simulink model "Final_Battery_model (1)"  (R2023b)
settings: Solver=VariableStepAuto  StartTime=0.0  StopTime=inf  FixedStep=1  RelTol=1e-5
undefined symbols (not defined in the file): C
settings Model: PacingRate=100  Creator=vahid  LastModifiedBy=vahid
settings SolverCC: ZeroCrossAlgorithm=Adaptive
settings OptimizationCC: BlockReduction=off  DefaultParameterBehavior=Inlined  BufferReuse=off
settings DebuggingCC: IgnoredZcDiagnostic=none

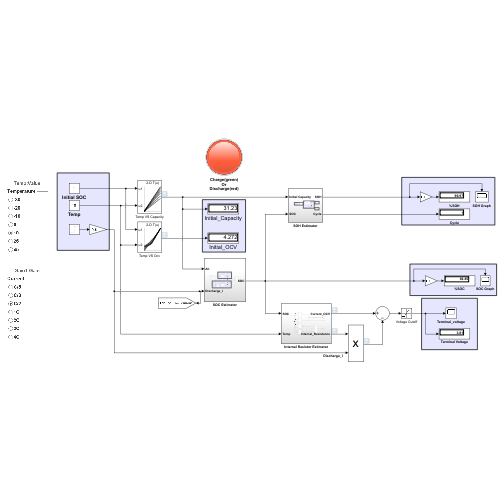
[thumbnail: Simulink's stored preview of the top-level diagram]
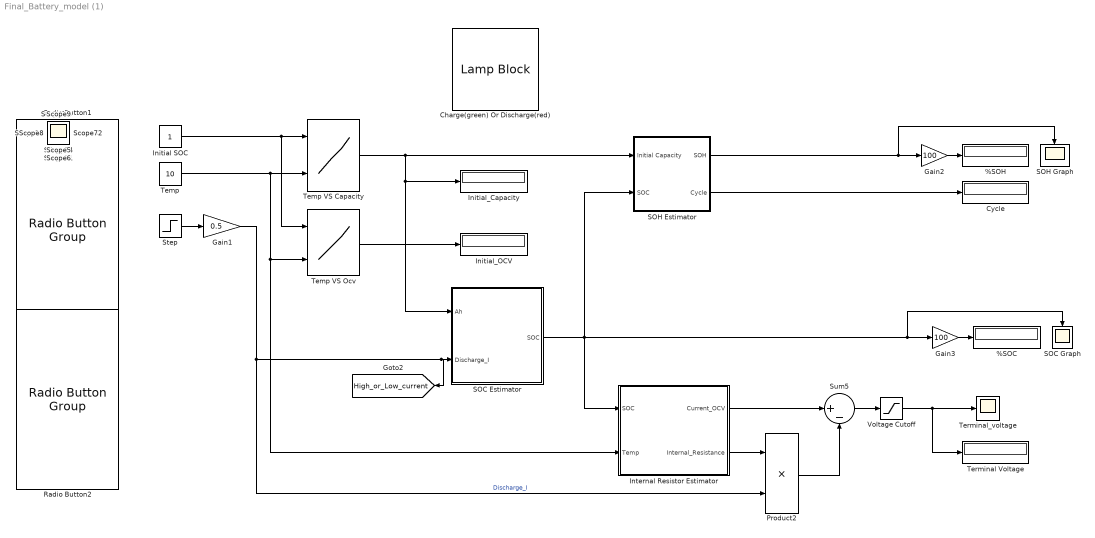
== system Final_Battery_model (1) ==
  %SOC : Display
  %SOH : Display
  Charge(green) Or Discharge(red) : LampBlock  LabelPosition=Hide
  Cycle : Display
  Gain1 : Gain  Gain=0.5
  Gain2 : Gain  Gain=100
  Gain3 : Gain  Gain=100
  Initial SOC : Constant  SampleTime=1
  Initial_Capacity : Display
  Initial_OCV : Display
  Internal Resistor Estimator : Subsystem
  Product2 : Product
  Radio Button1 : RadioButtonGroup  SelectedLabel=10  ButtonGroupName=Temperature
      settings: Values={{'-30', '-20', '-10', '0', '10', '25', '45'}, [-30 -20 -10 0 10 25 45]}
  Radio Button2 : RadioButtonGroup  SelectedLabel=C/2  ButtonGroupName=Current
      settings: Values={{'C/5', 'C/3', 'C/2', '1C', '2C', '3C', '4C'}, [0.2 0.33 0.5 1 2 3 4]}
  SOC Estimator : Subsystem
  SOC Graph : Scope
  SOH Estimator : Subsystem
  SOH Graph : Scope
  Step : Step  Before=32  After=32  SampleTime=0
  Sum5 : Sum  Inputs=|+-
  Temp : Constant  Value=10
  Temp VS Capacity : Lookup_n-D  BreakpointsForDimension1=[0.05;0.1;0.2;0.3;0.4;0.5;0.6;0.7;0.8;0.9;1]  BreakpointsForDimension2=[-30;-20;-10;0;10;25;45;55]  Table=[0.9696 1.142325 1.332525 1.44755 1.561325 1.666425 1.751575 1.7742;1.9392 2.28465 2.66505 2.8951 3.12265 3.33285 3.50315 3.5484;3.8784 4.5693 5.3301 5.7902 6.2453 6.6657 7.0063 7.0968;5.8176 6.85395 7.99515 8.6853 9.36795 9.99855 10.50945 10.6452;7.7568 9.1386 10.6602 11.5804 12.4906 13.3314 14.0126 14.1936;9.696 11.42325 13.32525 14.4755 15.61325 16.66425 17.51575 17.742;11.6352 13.7079 15.9903 17.3706 18.7359 19.9971 21.0189 21.2904;13.5744 15.99255 18.65535 20.2657 21.85855 23.32995 24.52205 24.8388;15.5136 18.2772 21.3204 23.1608 24.9812 26.6628 28.0252 28.3872;17.4528 20.56185 23.98545 26.0559 28.10385 29.99565 31.52835 31.9356;19.392 22.8465 26.6505 28.951 31.2265 33.3285 35.0315 35.484]  InternalRulePriority=Speed  RndMeth=Simplest
      settings: InputPortMap=u0,u1
  Temp VS Ocv : Lookup_n-D  BreakpointsForDimension1=[0.05;0.1;0.2;0.3;0.4;0.5;0.6;0.7;0.8;0.9;1]  BreakpointsForDimension2=[-30;-20;-10;0;10;25;45;55]  Table=[3.631 3.597 3.574 3.559 3.523 3.473 3.473 3.425;3.635 3.61 3.588 3.581 3.558 3.516 3.516 3.462;3.669 3.647 3.625 3.617 3.608 3.589 3.589 3.547;3.713 3.69 3.663 3.651 3.641 3.632 3.632 3.619;3.768 3.749 3.715 3.694 3.678 3.665 3.665 3.655;3.831 3.821 3.788 3.764 3.743 3.72 3.72 3.702;3.898 3.901 3.878 3.862 3.85 3.831 3.831 3.806;3.971 3.984 3.973 3.968 3.957 3.938 3.938 3.917;4.048 4.071 4.069 4.07 4.063 4.05 4.05 4.033;4.133 4.154 4.158 4.165 4.164 4.161 4.161 4.149;4.266 4.268 4.266 4.272 4.272 4.278 4.278 4.261]  InternalRulePriority=Speed  RndMeth=Simplest
      settings: InputPortMap=u0,u1
  Terminal Voltage : Display
  Terminal_voltage : Scope
  Voltage Cutoff : Saturate  UpperLimit=4.3  LowerLimit=2.7
  Scope{,2..15} (15 alike) : Scope
  tag scope: High_or_Low_current=global
  wires:
  Temp VS Capacity/1 -> SOH Estimator/1(Initial Capacity), Initial_Capacity/1, SOC Estimator/1(Ah)
  Temp VS Ocv/1 -> Initial_OCV/1
  Initial SOC/1 -> Temp VS Ocv/1, Temp VS Capacity/1
  Temp/1 -> Internal Resistor Estimator/2(Temp), Temp VS Ocv/2, Temp VS Capacity/2
  Product2/1 -> Sum5/2
  Internal Resistor Estimator/1(Current_OCV) -> Sum5/1
  Internal Resistor Estimator/2(Internal_Resistance) -> Product2/1
  Step/1 -> Gain1/1
  Gain1/1 -> [High_or_Low_current], SOC Estimator/2(Discharge_I), Product2/2  "Discharge_I"
  Sum5/1 -> Voltage Cutoff/1
  SOH Estimator/1(SOH) -> SOH Graph/1, Gain2/1
  Gain2/1 -> %SOH/1
  SOH Estimator/2(Cycle) -> Cycle/1
  SOC Estimator/1(SOC) -> Internal Resistor Estimator/1(SOC), Gain3/1, SOC Graph/1, SOH Estimator/2(SOC)
  Voltage Cutoff/1 -> Terminal Voltage/1, Terminal_voltage/1
  Gain3/1 -> %SOC/1

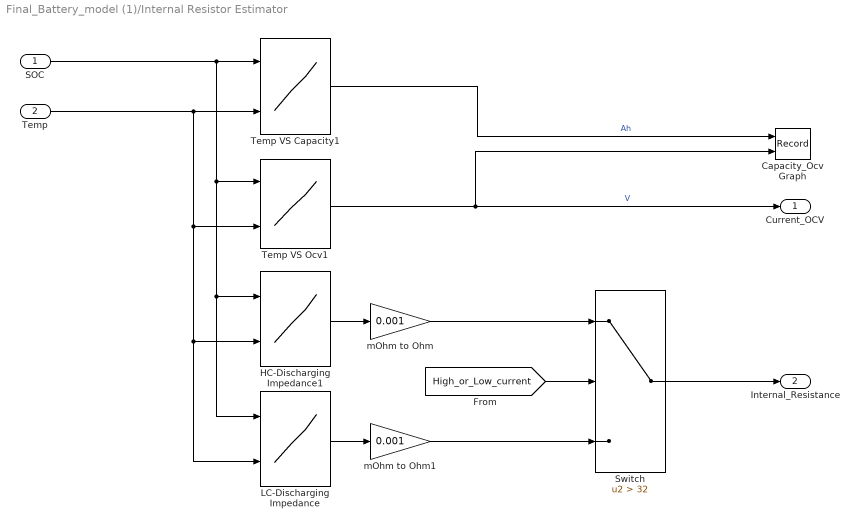
== system Final_Battery_model (1)/Internal Resistor Estimator ==
  SOC : Inport
  Temp : Inport  Port=2
  Capacity_Ocv Graph : Record  FileSettingsInternal="{\"entries\":[{\"content\":{\"excelSettings\":{\"content\":{},\"type\":\"Streamout.ExcelSettings\"}},\"type\":\"Streamout.FileSettingStorage\",\"uuid\":\"\"}],\"packageUris\":[\"http:\\/\\/schema.mathworks.com\\/mf0\\/streamout_blocks\\/R2020a\"],\"version\":\"1.0\"}"  Layout=[1 1]  SignalsInternal="{\"entries\":[{\"content\":{\"signals\":[{\"content\":{\"blockPath\":[],\"dimensions\":[1],\"domain\":\"\",\"lineColor\":\"#a2142f\",\"plots\":[1],\"port\":1,\"signalID\":7779,\"signalName\":\"XY Graph:1\"},\"type\":\"RecordBlkView.Signal\",\"uuid\":\"\"},{\"content\":{\"blockPath\":[],\"dimensions\":[1],\"domain\":\"\",\"lineColor\":\"#139fff\",\"plots\":[1],\"port\":2,\"signalID\":7782,\"signalName\":\"XY Graph:2\"},\"type\":\"RecordBlkView.Signal\",\"uuid\":\"\"}]},\"type\":\"RecordBlkView.InputSignals\",\"uuid\":\"\"}],\"packageUris\":[\"http:\\/\\/schema.mathworks.com\\/mf0\\/streamout_blocks\\/R2020a\"],\"version\":\"1.0\"}"  VisualizationBindings="{\"xyplotplugin\":{\"info\":[{\"series\":[{\"bindingParametersList\":[{\"parameter\":\"X-Axis\",\"signalID\":7779,\"signalName\":\"XY Graph:1\"},{\"parameter\":\"Y-Axis\",\"signalID\":7782,\"signalName\":\"XY Graph:2\"}],\"seriesID\":9451}],\"subplotID\":1}]}}"  CompatibilityTag=XY
  HC-Discharging Impedance1 : Lookup_n-D  BreakpointsForDimension1=[0;0.05;0.1;0.2;0.3;0.4;0.5;0.6;0.7;0.8;0.9;1]  BreakpointsForDimension2=[-30;-20;-10;0;10;25;45;55]  Table=[75.5 51.2 28.1 17.5 14.1 8.88 5.49 4.87;75.5 51.2 28.1 17.5 14.1 8.88 5.49 4.87;69.9 45.3 24.1 14.2 10.3 7.3 3.2 4.2;61.2 35.8 17.8 10 6.1 4.3 3.5 2.3;47.7 26.6 13.8 8.1 5.1 4 3 2;37.1 23.5 11.7 7.4 4.8 3.7 3 1.9;30.5 21.4 10.6 7.1 4.7 3.9 2.2 1.7;27.5 18.3 10 7 4.7 3.9 2.1 1.7;24.8 16.7 9.7 6.9 4.7 4 2.2 1.9;22.9 16.1 9.5 6.9 4.8 4 2.3 1.9;22.1 15.8 9.5 7 4.9 4.1 2.3 1.9;22.4 16.7 9.7 7.3 5.1 3.9 2.2 1.8]  InternalRulePriority=Speed  RndMeth=Simplest
      settings: InputPortMap=u0,u1
  LC-Discharging Impedance : Lookup_n-D  BreakpointsForDimension1=[0;0.05;0.1;0.15;0.2;0.25;0.3;0.35;0.4;0.45;0.5;0.55;0.6;0.65;0.7;0.75;0.8;0.85;0.9;0.95;1]  BreakpointsForDimension2=[-30;-20;-10;0;10;25;45]  Table=[124.53 60.78 33.59 13.67 8.39 4.69 3.13;124.53 60.78 33.59 13.67 8.39 4.69 3.13;122.03 59.69 32.5 12.61 7.28 3.91 2.34;119.84 58.59 31.88 11.97 6.78 3.44 2.03;119.38 57.5 30.94 11.54 6.51 3.28 1.87;118.59 56.41 30.31 11.27 6.32 3.28 1.88;117.97 55.78 29.84 11.17 6.2 2.97 1.87;117.34 55.63 29.53 11.05 6.13 3.13 1.88;117.03 55.63 29.38 11.08 6.22 3.12 1.72;116.88 55.62 29.53 11.22 6.3 3.28 1.88;116.72 55.78 29.69 11.51 6.49 3.28 1.88;117.03 55.78 30 11.78 6.75 3.59 2.03;117.19 55.94 30 12.04 7.14 3.91 2.19;117.34 56.41 30.16 12.21 7.11 3.75 2.19;118.28 57.03 30.47 12.3 7.09 3.75 2.19;119.53 57.81 30.94 12.42 7.09 3.91 2.19;121.56 59.06 31.25 12.42 7.18 3.59 2.19;124.38 60.47 31.88 12.52 7.19 3.75 2.03;128.59 62.97 32.97 12.78 7.23 3.44 2.03;136.09 67.81 35.78 13.58 7.67 3.75 2.03;155 80.94 43.91 16.29 9.06 3.91 2.34]  InternalRulePriority=Speed  RndMeth=Simplest
      settings: InputPortMap=u0,u1
  Switch : Switch  Criteria=u2 > Threshold  Threshold=32  SaturateOnIntegerOverflow=off  InputSameDT=off
  Temp VS Capacity1 : Lookup_n-D  BreakpointsForDimension1=[0.05;0.1;0.2;0.3;0.4;0.5;0.6;0.7;0.8;0.9;1]  BreakpointsForDimension2=[-30;-20;-10;0;10;25;45;55]  Table=[0.9696 1.142325 1.332525 1.44755 1.561325 1.666425 1.751575 1.7742;1.9392 2.28465 2.66505 2.8951 3.12265 3.33285 3.50315 3.5484;3.8784 4.5693 5.3301 5.7902 6.2453 6.6657 7.0063 7.0968;5.8176 6.85395 7.99515 8.6853 9.36795 9.99855 10.50945 10.6452;7.7568 9.1386 10.6602 11.5804 12.4906 13.3314 14.0126 14.1936;9.696 11.42325 13.32525 14.4755 15.61325 16.66425 17.51575 17.742;11.6352 13.7079 15.9903 17.3706 18.7359 19.9971 21.0189 21.2904;13.5744 15.99255 18.65535 20.2657 21.85855 23.32995 24.52205 24.8388;15.5136 18.2772 21.3204 23.1608 24.9812 26.6628 28.0252 28.3872;17.4528 20.56185 23.98545 26.0559 28.10385 29.99565 31.52835 31.9356;19.392 22.8465 26.6505 28.951 31.2265 33.3285 35.0315 35.484]  InternalRulePriority=Speed  RndMeth=Simplest
      settings: InputPortMap=u0,u1
  Temp VS Ocv1 : Lookup_n-D  BreakpointsForDimension1=[0;0.05;0.1;0.2;0.3;0.4;0.5;0.6;0.7;0.8;0.9;1]  BreakpointsForDimension2=[-30;-20;-10;0;10;25;45;55]  Table=[2.7 2.7 2.7 2.7 2.7 2.7 2.7 2.7;3.631 3.597 3.574 3.559 3.523 3.473 3.473 3.425;3.635 3.61 3.588 3.581 3.558 3.516 3.516 3.462;3.669 3.647 3.625 3.617 3.608 3.589 3.589 3.547;3.713 3.69 3.663 3.651 3.641 3.632 3.632 3.619;3.768 3.749 3.715 3.694 3.678 3.665 3.665 3.655;3.831 3.821 3.788 3.764 3.743 3.72 3.72 3.702;3.898 3.901 3.878 3.862 3.85 3.831 3.831 3.806;3.971 3.984 3.973 3.968 3.957 3.938 3.938 3.917;4.048 4.071 4.069 4.07 4.063 4.05 4.05 4.033;4.133 4.154 4.158 4.165 4.164 4.161 4.161 4.149;4.266 4.268 4.266 4.272 4.272 4.278 4.278 4.261]  InternalRulePriority=Speed  RndMeth=Simplest
      settings: InputPortMap=u0,u1
  mOhm to Ohm : Gain  Gain=0.001
  mOhm to Ohm1 : Gain  Gain=0.001
  Current_OCV : Outport
  Internal_Resistance : Outport  Port=2
  wires:
  HC-Discharging Impedance1/1 -> mOhm to Ohm/1
  Temp VS Ocv1/1 -> Capacity_Ocv Graph/2, Current_OCV/1  "V"
  SOC/1 -> Temp VS Ocv1/1, HC-Discharging Impedance1/1, LC-Discharging Impedance/1, Temp VS Capacity1/1
  LC-Discharging Impedance/1 -> mOhm to Ohm1/1
  Temp/1 -> Temp VS Ocv1/2, HC-Discharging Impedance1/2, LC-Discharging Impedance/2, Temp VS Capacity1/2
  [High_or_Low_current] -> Switch/2
  mOhm to Ohm1/1 -> Switch/3
  Switch/1 -> Internal_Resistance/1
  mOhm to Ohm/1 -> Switch/1
  Temp VS Capacity1/1 -> Capacity_Ocv Graph/1  "Ah"

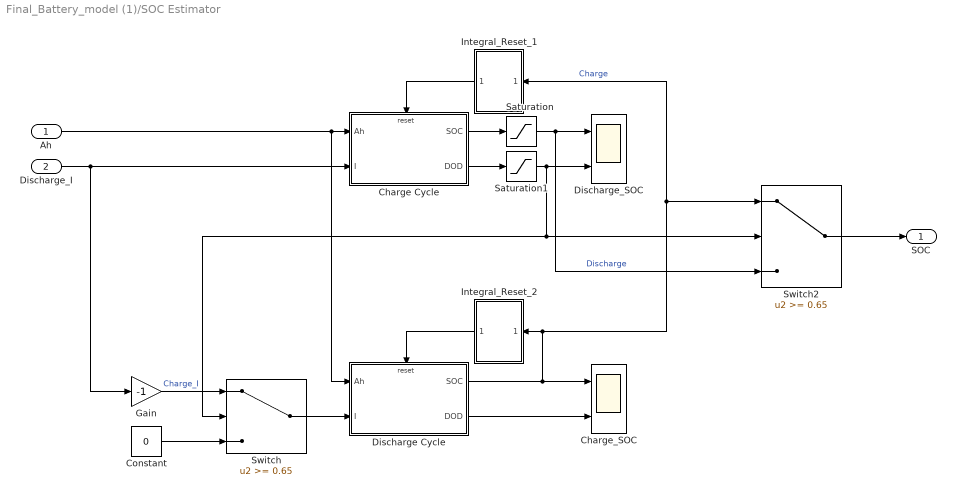
== system Final_Battery_model (1)/SOC Estimator ==
  Ah : Inport
  Discharge_I : Inport  Port=2
  Charge Cycle : Subsystem  TreatAsAtomicUnit=on
  Charge_SOC : Scope  NumInputPorts=2
  Constant : Constant  Value=0
  Discharge Cycle : Subsystem  TreatAsAtomicUnit=on
  Discharge_SOC : Scope  NumInputPorts=2
  Gain : Gain  Gain=-1
  Integral_Reset_1 : Subsystem
  Integral_Reset_2 : Subsystem
  Saturation : Saturate  UpperLimit=1  LowerLimit=0.35
  Saturation1 : Saturate  UpperLimit=0.65  LowerLimit=0
  Switch : Switch  Threshold=0.65  SaturateOnIntegerOverflow=off  InputSameDT=off
  Switch2 : Switch  Threshold=0.65  SaturateOnIntegerOverflow=off  InputSameDT=off
  SOC : Outport
  wires:
  Ah/1 -> Charge Cycle/1(Ah), Discharge Cycle/1(Ah)
  Discharge Cycle/2(DOD) -> Charge_SOC/2
  Saturation/1 -> Switch2/3, Discharge_SOC/1  "Discharge"
  Discharge Cycle/1(SOC) -> Charge_SOC/1, Integral_Reset_1/1(SOC), Switch2/1, Integral_Reset_2/1(SOC)  "Charge"
  Discharge_I/1 -> Charge Cycle/2(I), Gain/1
  Integral_Reset_1/1(Out1) -> Charge Cycle/Reset
  Charge Cycle/2(DOD) -> Saturation1/1
  Switch/1 -> Discharge Cycle/2(I)
  Integral_Reset_2/1(Out1) -> Discharge Cycle/Reset
  Saturation1/1 -> Switch2/2, Switch/2, Discharge_SOC/2
  Gain/1 -> Switch/1  "Charge_I"
  Charge Cycle/1(SOC) -> Saturation/1
  Constant/1 -> Switch/3
  Switch2/1 -> SOC/1

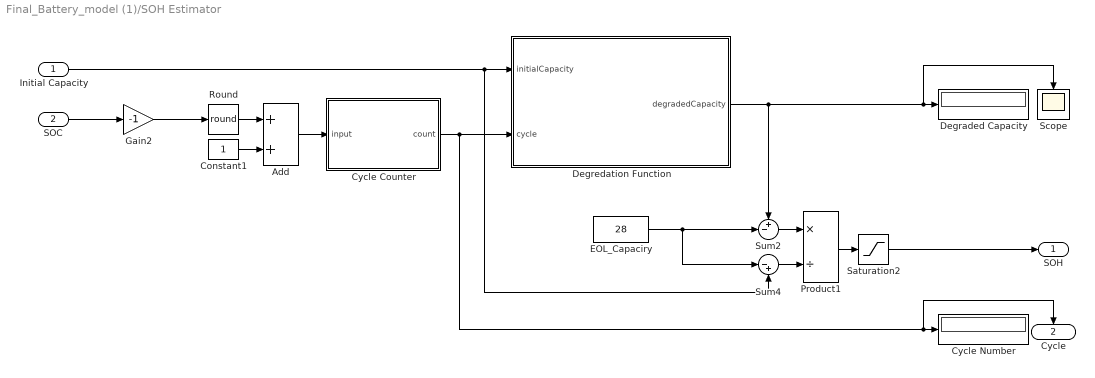
== system Final_Battery_model (1)/SOH Estimator ==
  Initial Capacity : Inport
  SOC : Inport  Port=2
  Add : Sum
  Constant1 : Constant
  Cycle Counter : MATLAB Function  TreatAsAtomicUnit=on
  Cycle Number : Display
  Degraded Capacity : Display
  Degredation Function : MATLAB Function  TreatAsAtomicUnit=on
  EOL_Capaciry : Constant  Value=28
  Gain2 : Gain  Gain=-1
  Product1 : Product  Inputs=*/
  Round : Rounding  Operator=round
  Saturation2 : Saturate  UpperLimit=1  LowerLimit=0
  Scope : Scope
  Sum2 : Sum  Inputs=+-|
  Sum4 : Sum  Inputs=|-+
  SOH : Outport
  Cycle : Outport  Port=2
  wires:
  Gain2/1 -> Round/1
  Sum2/1 -> Product1/1
  Cycle Counter/1(count) -> Cycle/1, Cycle Number/1, Degredation Function/2(cycle)
  Degredation Function/1(degradedCapacity) -> Sum2/1, Scope/1, Degraded Capacity/1
  Round/1 -> Add/1
  EOL_Capaciry/1 -> Sum2/2, Sum4/1
  Saturation2/1 -> SOH/1
  Constant1/1 -> Add/2
  Sum4/1 -> Product1/2
  Initial Capacity/1 -> Sum4/2, Degredation Function/1(initialCapacity)
  Product1/1 -> Saturation2/1
  Add/1 -> Cycle Counter/1(input)
  SOC/1 -> Gain2/1

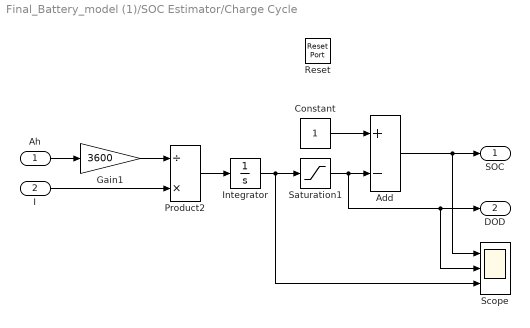
== system Final_Battery_model (1)/SOC Estimator/Charge Cycle ==
  Ah : Inport
  I : Inport  Port=2
  Reset : ResetPort  DisableCoverage=on
  Add : Sum  Inputs=+-
  Constant : Constant
  Gain1 : Gain  Gain=3600
  Integrator : Integrator
  Product2 : Product  Inputs=/*
  Saturation1 : Saturate  UpperLimit=1  LowerLimit=0
  Scope : Scope  NumInputPorts=3
  SOC : Outport
  DOD : Outport  Port=2
  wires:
  Constant/1 -> Add/1
  Product2/1 -> Integrator/1
  Ah/1 -> Gain1/1
  Add/1 -> SOC/1, Scope/1
  Saturation1/1 -> Add/2, Scope/2, DOD/1
  Integrator/1 -> Saturation1/1, Scope/3
  Gain1/1 -> Product2/1
  I/1 -> Product2/2

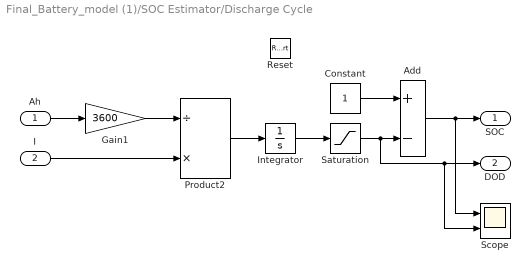
== system Final_Battery_model (1)/SOC Estimator/Discharge Cycle ==
  Ah : Inport
  I : Inport  Port=2
  Reset : ResetPort  DisableCoverage=on
  Add : Sum  Inputs=+-
  Constant : Constant
  Gain1 : Gain  Gain=3600
  Integrator : Integrator  InitialCondition=0.65
  Product2 : Product  Inputs=/*
  Saturation : Saturate  UpperLimit=1  LowerLimit=0
  Scope : Scope  NumInputPorts=2
  SOC : Outport
  DOD : Outport  Port=2
  wires:
  Ah/1 -> Gain1/1
  Product2/1 -> Integrator/1
  Integrator/1 -> Saturation/1
  Gain1/1 -> Product2/1
  I/1 -> Product2/2
  Add/1 -> Scope/1, SOC/1
  Saturation/1 -> Scope/2, DOD/1, Add/2
  Constant/1 -> Add/1

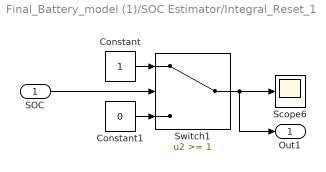
== system Final_Battery_model (1)/SOC Estimator/Integral_Reset_1 ==
  SOC : Inport
  Constant : Constant
  Constant1 : Constant  Value=0
  Scope6 : Scope
  Switch1 : Switch  Threshold=1  SaturateOnIntegerOverflow=off  InputSameDT=off
  Out1 : Outport
  wires:
  Switch1/1 -> Scope6/1, Out1/1
  SOC/1 -> Switch1/2
  Constant1/1 -> Switch1/3
  Constant/1 -> Switch1/1

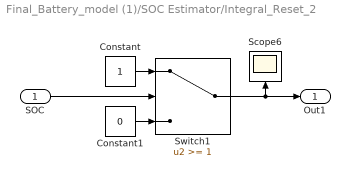
== system Final_Battery_model (1)/SOC Estimator/Integral_Reset_2 ==
  SOC : Inport
  Constant : Constant
  Constant1 : Constant  Value=0
  Scope6 : Scope
  Switch1 : Switch  Threshold=1  SaturateOnIntegerOverflow=off  InputSameDT=off
  Out1 : Outport
  wires:
  Constant/1 -> Switch1/1
  Constant1/1 -> Switch1/3
  SOC/1 -> Switch1/2
  Switch1/1 -> Out1/1, Scope6/1

== matlab function Final_Battery_model (1)/SOH Estimator/Degredation Function ==
  data: initialCapacity input; cycle input; degradedCapacity output
function degradedCapacity = capacity_fade(initialCapacity, cycle)

    % Constants
    degradationRate = 0.001;  % Capacity degradation rate per hour
     
    % Capacity fade model (linear degradation)
    degradedCapacity = initialCapacity - degradationRate * cycle;

end

== matlab function Final_Battery_model (1)/SOH Estimator/Cycle Counter ==
  settings: updateMethod=DISCRETE
  data: input input; count output
function count = countOnRisingEdge(input)
    persistent prevInput;
    persistent totalCount;
    
    if isempty(prevInput)
        prevInput = 0;
    end
    
    if isempty(totalCount)
        totalCount = 0;
    end
    
    % Detect rising edge
    if input == 1 && prevInput == 0
        totalCount = totalCount + 1;
    end
    
    % Save the current input for the next iteration
    prevInput = input;
    
    % Output the total count
    count = totalCount;
end
